simulink model "Integral_Control"  (R2021b)
settings: Solver=VariableStepAuto  StartTime=0.0  StopTime=100  RelTol=1e-3
undefined symbols (not defined in the file or in its folder): A, B, C, K1, K2
settings Model: Creator=parsiz  LastModifiedBy=Asus
settings SolverCC: AlgebraicLoopSolver=TrustRegion
settings DataIOCC: ReturnWorkspaceOutputs=off
settings DebuggingCC: SFMachineParentedDataDiag=warning  ArithmeticOperatorsInVariantConditions=warning
settings SFSimCC: SimUseLocalCustomCode=off  CustomCodeUndefinedFunction=UseInterfaceOnly
settings RTWCC: RTWUseLocalCustomCode=off
settings CodeAppCC: StateflowObjectComments=on

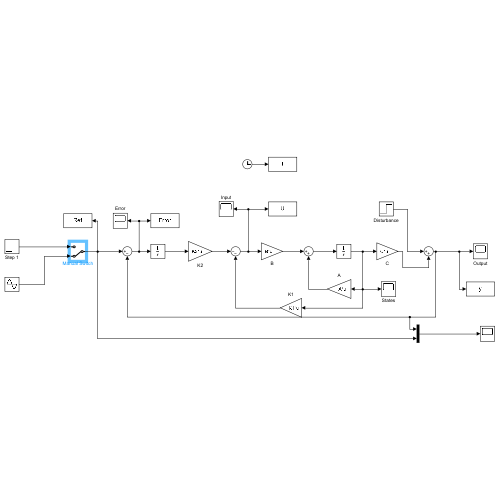
[thumbnail: Simulink's stored preview of the top-level diagram]
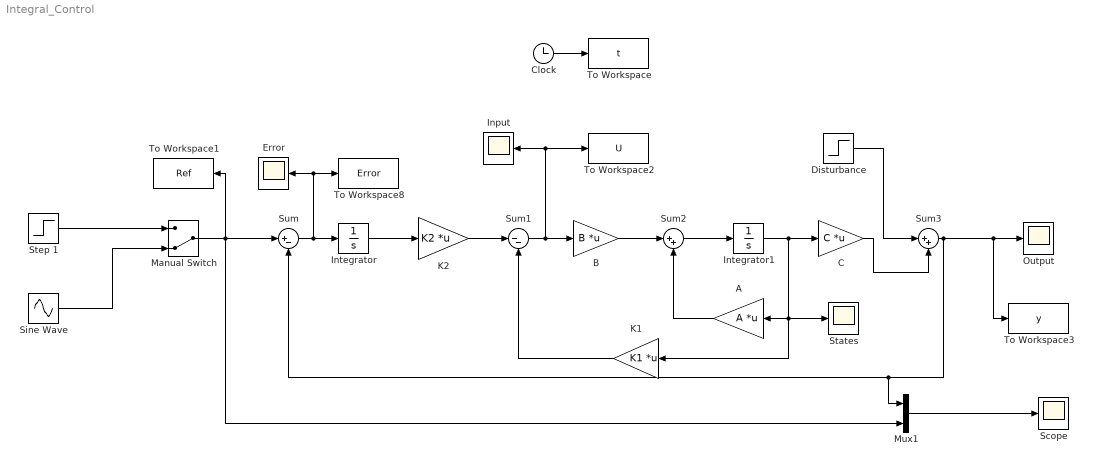
== system Integral_Control ==
  A : Gain  Gain=A  Multiplication=Matrix(K*u)
  B : Gain  Gain=B  Multiplication=Matrix(K*u)
  C : Gain  Gain=C  Multiplication=Matrix(K*u)
  Clock : Clock
  Disturbance : Step  Time=20  After=0  SampleTime=0
  Error : Scope
  Input : Scope
  Integrator : Integrator
  Integrator1 : Integrator
  K1 : Gain  Gain=K1  Multiplication=Matrix(K*u)
  K2 : Gain  Gain=K2  Multiplication=Matrix(K*u)
  Manual Switch : ManualSwitch  CurrentSetting=0
  Mux1 : Mux  Inputs=2
  Output : Scope
  Scope : Scope
  Sine Wave : Sin  SampleTime=0
  States : Scope
  Step 1 : Step  After=10  SampleTime=0.001
  Sum : Sum  Inputs=|+-
  Sum1 : Sum  Inputs=|--
  Sum2 : Sum  Inputs=|++
  Sum3 : Sum  Inputs=|++
  To Workspace : ToWorkspace  VariableName=t  SaveFormat=Timeseries  SampleTime=-1
  To Workspace1 : ToWorkspace  VariableName=Ref  SaveFormat=Timeseries  SampleTime=-1
  To Workspace2 : ToWorkspace  VariableName=U  SaveFormat=Timeseries  SampleTime=-1
  To Workspace3 : ToWorkspace  VariableName=y  SaveFormat=Timeseries  SampleTime=-1
  To Workspace8 : ToWorkspace  VariableName=Error  SaveFormat=Timeseries  SampleTime=-1
  wires:
  Clock/1 -> To Workspace/1
  Step 1/1 -> Manual Switch/1
  Sum/1 -> Integrator/1, To Workspace8/1, Error/1
  Integrator/1 -> K2/1
  K2/1 -> Sum1/1
  B/1 -> Sum2/1
  Sum2/1 -> Integrator1/1
  Integrator1/1 -> K1/1, States/1, A/1, C/1
  A/1 -> Sum2/2
  K1/1 -> Sum1/2
  Mux1/1 -> Scope/1
  Sum1/1 -> Input/1, To Workspace2/1, B/1
  Sine Wave/1 -> Manual Switch/2
  Manual Switch/1 -> Mux1/2, Sum/1, To Workspace1/1
  Disturbance/1 -> Sum3/1
  C/1 -> Sum3/2
  Sum3/1 -> Mux1/1, Sum/2, To Workspace3/1, Output/1
